simulink subsystem "Logging_Metrics"  (R2025a)
settings: Solver=VariableStepAuto  StartTime=0.0  StopTime=10.0  RelTol=1e-3
settings Model: Creator=Jackt  LastModifiedBy=Jackt

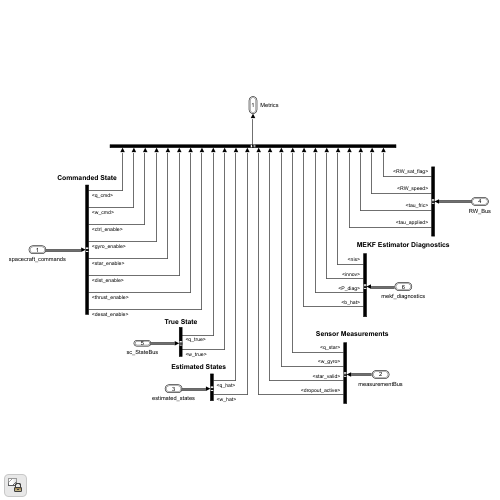
[thumbnail: Simulink's stored preview of the top-level diagram]
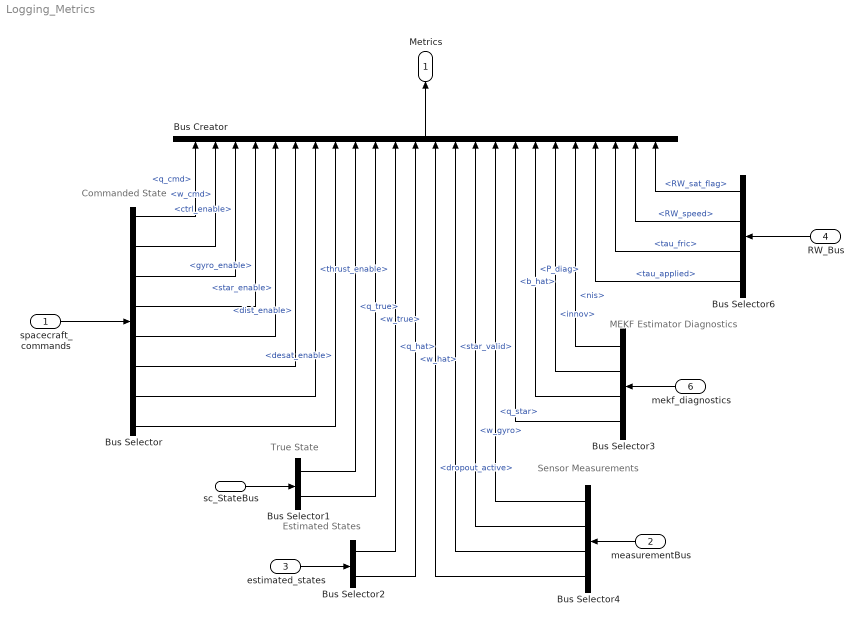
== system Logging_Metrics ==
  note: MEKF Estimator Diagnostics
  note: Sensor Measurements
  note: Estimated States
  note: True State
  note: Commanded State
  spacecraft_commands : Inport  OutDataTypeStr=Bus: commandBus
  measurementBus : Inport  Port=2  OutDataTypeStr=Bus: measurementBus
  estimated_states : Inport  Port=3  OutDataTypeStr=Bus: estimatedStateBus
  RW_Bus : Inport  Port=4  OutDataTypeStr=Bus: reactionWheelBus
  sc_StateBus : Inport  Port=5  OutDataTypeStr=Bus: sc_stateBus
  mekf_diagnostics : Inport  Port=6  OutDataTypeStr=Bus: mekf_diagnostics
  Bus Creator : BusCreator  Inputs=24
  Bus Selector : BusSelector  OutputSignals=q_cmd,w_cmd,ctrl_enable,gyro_enable,star_enable,dist_enable,thrust_enable,desat_enable
  Bus Selector1 : BusSelector  OutputSignals=q_true,w_true
  Bus Selector2 : BusSelector  OutputSignals=q_hat,w_hat
  Bus Selector3 : BusSelector  OutputSignals=nis,innov,P_diag,b_hat
  Bus Selector4 : BusSelector  OutputSignals=q_star,w_gyro,star_valid,dropout_active
  Bus Selector6 : BusSelector  OutputSignals=RW_sat_flag,RW_speed,tau_fric,tau_applied
  Metrics : Outport  OutDataTypeStr=Bus: metrics
  wires:
  spacecraft_commands/1 -> Bus Selector/1
  Bus Selector/1 -> Bus Creator/1  "<q_cmd>"
  Bus Selector/2 -> Bus Creator/2  "<w_cmd>"
  Bus Selector/3 -> Bus Creator/3  "<ctrl_enable>"
  Bus Selector/4 -> Bus Creator/4  "<gyro_enable>"
  Bus Selector/5 -> Bus Creator/5  "<star_enable>"
  Bus Selector/6 -> Bus Creator/6  "<dist_enable>"
  Bus Selector/7 -> Bus Creator/7  "<thrust_enable>"
  Bus Selector/8 -> Bus Creator/8  "<desat_enable>"
  sc_StateBus/1 -> Bus Selector1/1
  Bus Selector1/2 -> Bus Creator/10  "<w_true>"
  Bus Selector1/1 -> Bus Creator/9  "<q_true>"
  estimated_states/1 -> Bus Selector2/1
  Bus Selector2/1 -> Bus Creator/11  "<q_hat>"
  Bus Selector2/2 -> Bus Creator/12  "<w_hat>"
  mekf_diagnostics/1 -> Bus Selector3/1
  Bus Selector3/4 -> Bus Creator/17  "<b_hat>"
  Bus Selector3/1 -> Bus Creator/20  "<nis>"
  Bus Selector3/3 -> Bus Creator/18  "<P_diag>"
  Bus Selector3/2 -> Bus Creator/19  "<innov>"
  measurementBus/1 -> Bus Selector4/1
  Bus Selector4/3 -> Bus Creator/14  "<star_valid>"
  Bus Selector4/4 -> Bus Creator/13  "<dropout_active>"
  Bus Selector4/2 -> Bus Creator/15  "<w_gyro>"
  Bus Selector4/1 -> Bus Creator/16  "<q_star>"
  RW_Bus/1 -> Bus Selector6/1
  Bus Selector6/4 -> Bus Creator/21  "<tau_applied>"
  Bus Selector6/1 -> Bus Creator/24  "<RW_sat_flag>"
  Bus Selector6/2 -> Bus Creator/23  "<RW_speed>"
  Bus Selector6/3 -> Bus Creator/22  "<tau_fric>"
  Bus Creator/1 -> Metrics/1
